simulink model "ACC_ISR"  (R2021b)
settings: Solver=FixedStepAuto  StartTime=0.0  StopTime=inf  FixedStep=0.01  RelTol=1e-3  EnableMultiTasking=on
libraries: arduinolib x4, simulink x2, arduinosensorlib x1
settings Model: ExtModeTrigDuration=2  Creator=user  LastModifiedBy=user
settings OptimizationCC: EnhancedBackFolding=on  PassReuseOutputArgsAs=Individual arguments  ZeroExternalMemoryAtStartup=off  ZeroInternalMemoryAtStartup=off  MaxStackSize=64  OptimizeBlockOrder=speed  DifferentSizesBufferReuse=on  OptimizationCustomize=off  EfficientTunableParamExpr=on
settings DebuggingCC: ParameterTunabilityLossMsg=error
settings HardwareCC: ProdBitPerInt=16  ProdBitPerPointer=16  ProdBitPerSizeT=16  ProdBitPerPtrDiffT=16  ProdLargestAtomicFloat=None  ProdWordSize=8  ProdHWDeviceType=Atmel->AVR
settings SFSimCC: MATLABDynamicMemAlloc=off
settings RTWCC: Description=Embedded Coder  SystemTargetFile=ert.tlc  HardwareBoard=Arduino Mega 2560  TemplateMakefile=ert_default_tmf  Toolchain=Arduino AVR  BuildConfiguration=Faster Runs
settings CodeAppCC: ForceParamTrailComments=on  IgnoreCustomStorageClasses=off  OperatorAnnotations=on  SimulinkDataObjDesc=on  SFDataObjDesc=on  InsertBlockDesc=on
settings ERTTargetCC: SupportContinuousTime=on  SupportVariableSizeSignals=on  ExtModeTransport=3  ExtModeStaticAlloc=on  ExtModeStaticAllocSize=2048  ExtModeMexFile=ext_xcp  ExtModeIntrfLevel=Level2 - Open

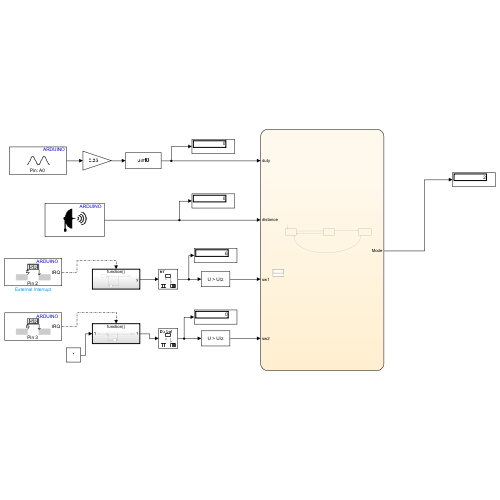
[thumbnail: Simulink's stored preview of the top-level diagram]
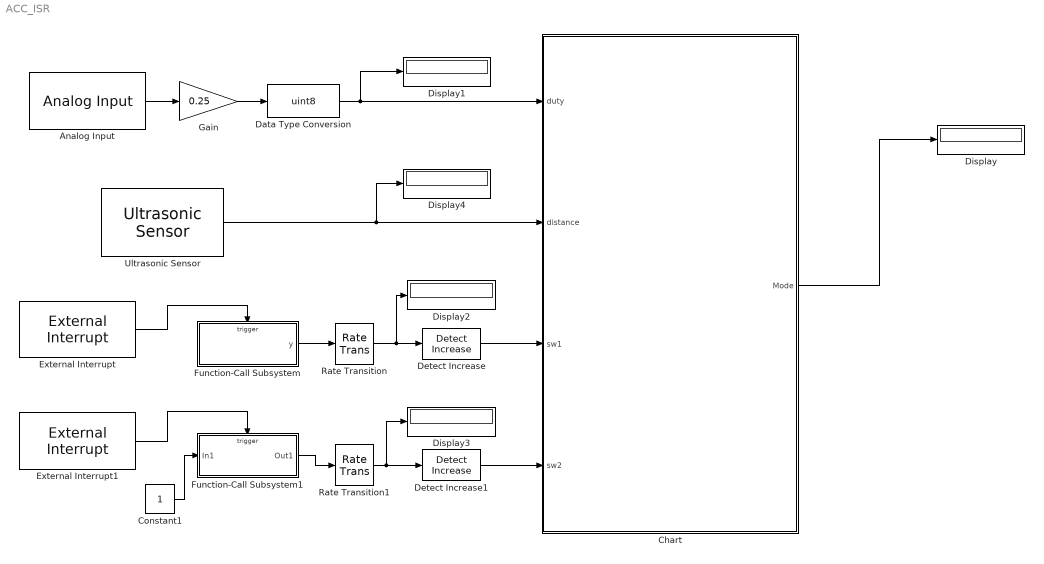
== system ACC_ISR ==
  Analog Input : arduinolib/Analog Input  pinNumber=0  ReadResultsOnly=off  ConversionTriggerSource=Software  ExternalTriggerType=uint32( 0 )  OutputDataType=uint16  EnableConversionCompleteNotify=off  EnableOuputStatus=off  SampleTime=-1  blockPlatform=arduino
  Chart : Stateflow chart  TreatAsAtomicUnit=on
      settings: PortSchema="{\"entries\":[{\"content\":{\"sides\":[{\"content\":{\"connectorIds\":[\"In3\",\"In4\",\"In1\",\"In2\"]},\"type\":\"ConnectorPlacement.EquallySpacedRectSide\",\"uuid\":\"ba3abb21-d0a5-4ef7-9df8-45f9f8fdbaa3\"},{\"content\":{\"connectorIds\":[\"Out1\"],\"side\":\"RIGHT\"},\"type\":\"ConnectorPlacement.EquallySpacedRectSide\",\"uuid\":\"4c869397-4c80-4d27-93b6-760fa6cdd1e5\"},{\"content\":{\"connectorIds\":[],\"side\":\"TOP\"},\"type\":\"ConnectorPlacement.EquallySpacedRectSide\",\"uuid\":\"e6ca1cf0-b515-4212-a22f-ac441a0348c8\"}]},\"type\":\"ConnectorPlacement.EquallySpacedConnector\",\"uuid\":\"bb3679c2-4e24-4074-9ab9-9aa27ac5c34d\"}],\"packageUris\":[\"http://schema.mathworks.com/mf0/Connector/R2020b\"],\"version\":\"1.0\"}"
  Constant1 : Constant
  Data Type Conversion : DataTypeConversion  OutDataTypeStr=uint8
  Detect Increase : simulink/Logic and Bit Operations/Detect Increase  vinit=0.0  OutDataTypeStr=boolean
  Detect Increase1 : simulink/Logic and Bit Operations/Detect Increase  vinit=0.0  OutDataTypeStr=uint8
  Display{,1..4} (5 alike) : Display
  External Interrupt : arduinolib/External Interrupt  Pin=2  PullUp=on  Mode=FALLING  InterruptSimulationInput=off
      settings: SourceProductBaseCode=ARDUINO
  External Interrupt1 : arduinolib/External Interrupt  Pin=3  PullUp=on  Mode=FALLING  InterruptSimulationInput=off
      settings: SourceProductBaseCode=ARDUINO
  Function-Call Subsystem : Subsystem  TreatAsAtomicUnit=on
  Function-Call Subsystem1 : Subsystem  TreatAsAtomicUnit=on
  Gain : Gain  Gain=0.25
  Rate Transition : RateTransition  Integrity=off  Deterministic=off
  Rate Transition1 : RateTransition  Deterministic=off
  Ultrasonic Sensor : arduinosensorlib/Ultrasonic Sensor  NumSignalPins=2  TrigPin=50  EchoPin=51  SignalPin=3  SampleTime_=0.1  blockPlatform=ARDUINO
      settings: SourceProductBaseCode=ARDUINO
  wires:
  Chart/1(Mode) -> Display/1
  External Interrupt/1 -> Function-Call Subsystem/Trigger
  Constant1/1 -> Function-Call Subsystem1/1(In1)
  External Interrupt1/1 -> Function-Call Subsystem1/Trigger
  Detect Increase1/1 -> Chart/2(sw2)
  Function-Call Subsystem/1(y) -> Rate Transition/1
  Function-Call Subsystem1/1(Out1) -> Rate Transition1/1
  Rate Transition1/1 -> Display3/1, Detect Increase1/1
  Rate Transition/1 -> Display2/1, Detect Increase/1
  Detect Increase/1 -> Chart/1(sw1)
  Analog Input/1 -> Gain/1
  Gain/1 -> Data Type Conversion/1
  Data Type Conversion/1 -> Display1/1, Chart/3(duty)
  Ultrasonic Sensor/1 -> Display4/1, Chart/4(distance)

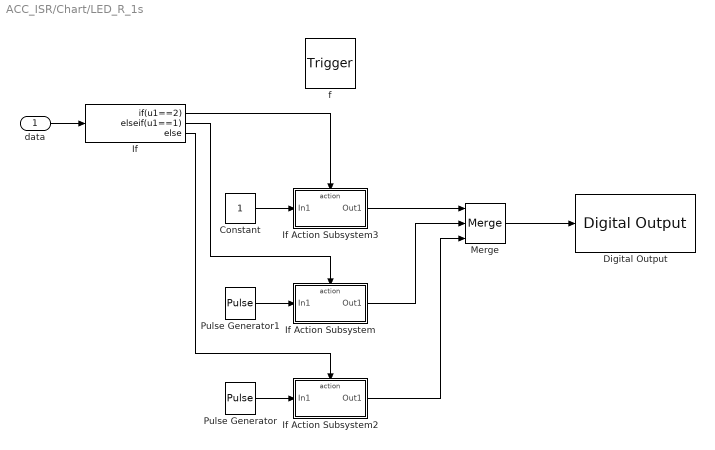
== system ACC_ISR/Chart/LED_R_1s ==
  data : Inport  OutDataTypeStr=double  PortDimensions=1
  f : TriggerPort  TriggerType=function-call  VariantControl=(inherit)
      settings: CopyFcn=Stateflow.SLINSF.SimulinkMan.removeBlockPreDeleteFcn  PreDeleteFcn=Stateflow.SLINSF.SimulinkMan.unsafePredeleteFcn
  Constant : Constant
  Digital Output : arduinolib/Digital Output  pinNumber=12  Direction=output  blockPlatform=arduino
  If : If  IfExpression=u1==2  ElseIfExpressions=u1==1
  If Action Subsystem : Subsystem  TreatAsAtomicUnit=on
  If Action Subsystem2 : Subsystem  TreatAsAtomicUnit=on
  If Action Subsystem3 : Subsystem  TreatAsAtomicUnit=on
  Merge : Merge  Inputs=3
  Pulse Generator : DiscretePulseGenerator  Period=200  PulseWidth=100  SampleTime=-1
  Pulse Generator1 : DiscretePulseGenerator  Period=40  PulseWidth=20  SampleTime=-1
  wires:
  data/1 -> If/1
  If/1 -> If Action Subsystem3/Action
  If/2 -> If Action Subsystem/Action
  If/3 -> If Action Subsystem2/Action
  Constant/1 -> If Action Subsystem3/1(In1)
  If Action Subsystem3/1(Out1) -> Merge/1
  Merge/1 -> Digital Output/1
  Pulse Generator1/1 -> If Action Subsystem/1(In1)
  If Action Subsystem/1(Out1) -> Merge/2
  Pulse Generator/1 -> If Action Subsystem2/1(In1)
  If Action Subsystem2/1(Out1) -> Merge/3

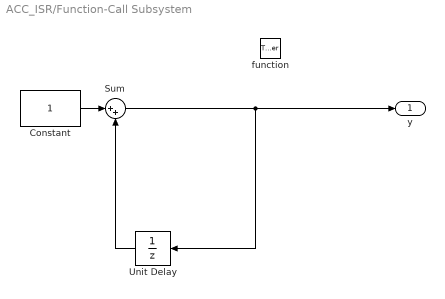
== system ACC_ISR/Function-Call Subsystem ==
  function : TriggerPort  TriggerType=function-call  VariantControl=(inherit)
  Constant : Constant
  Sum : Sum  Inputs=|++
  Unit Delay : UnitDelay  SampleTime=-1  HasFrameUpgradeWarning=on
  y : Outport
  wires:
  Unit Delay/1 -> Sum/2
  Constant/1 -> Sum/1
  Sum/1 -> Unit Delay/1, y/1

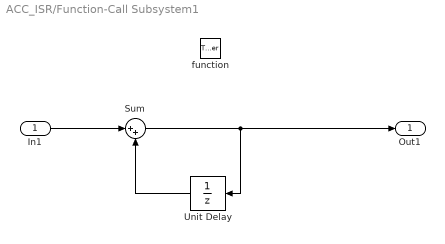
== system ACC_ISR/Function-Call Subsystem1 ==
  In1 : Inport
  function : TriggerPort  TriggerType=function-call  VariantControl=(inherit)
  Sum : Sum  Inputs=|++
  Unit Delay : UnitDelay  SampleTime=-1  HasFrameUpgradeWarning=on
  Out1 : Outport
  wires:
  Sum/1 -> Unit Delay/1, Out1/1
  Unit Delay/1 -> Sum/2
  In1/1 -> Sum/1

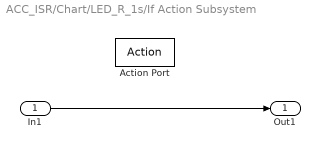
== system ACC_ISR/Chart/LED_R_1s/If Action Subsystem ==
  In1 : Inport
  Action Port : ActionPort  ActionPortLabel=elseif(u1==1)
  Out1 : Outport
  wires:
  In1/1 -> Out1/1

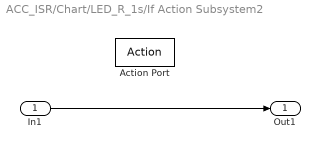
== system ACC_ISR/Chart/LED_R_1s/If Action Subsystem2 ==
  In1 : Inport
  Action Port : ActionPort  ActionPortLabel=else
  Out1 : Outport
  wires:
  In1/1 -> Out1/1

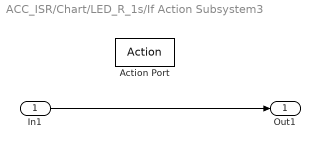
== system ACC_ISR/Chart/LED_R_1s/If Action Subsystem3 ==
  In1 : Inport
  Action Port : ActionPort  ActionPortLabel=if(u1==2)
  Out1 : Outport
  wires:
  In1/1 -> Out1/1

== stateflow chart ACC_ISR/Chart ==
  state ACC_off
    Mode=1;
    LED_R_1s(0);
  state ACC_standby
    Mode=2;
    LED_R_1s(1);
  state ACC_active
    Mode=3;
    LED_R_1s(2);
  state LED_R_1s(data) [function]
  (default) -> ACC_off
  ACC_standby -> ACC_active [order 2] : [sw1==1 ]
  ACC_off -> ACC_standby : [sw1==1 ]
  ACC_standby -> ACC_off [order 1] : [sw2==1]
  ACC_active -> ACC_off : [sw1 == 1 || sw2==1]
  data: data function_input double size=1; Mode output; sw1 input; sw2 input; duty input; distance input
